simulink model "Scenario_13_CoDeSys"  (R2012b)
settings: Solver=ode3  StartTime=0.0  StopTime=inf  FixedStep=Sample_Time_Model  RelTol=1e-3
PreLoadFcn:
  | Variablen_Scenario13
InitFcn:
  | BT = randperm(9);
values from neighbouring files (symbols this model uses):
  Band_Geschwindigkeit = 1.47    [Variablen_Scenario13.m]
  Band_Sensor_Hell_2_Z = -6.5    [Variablen_Scenario13.m]
  Band_Sensor_Hell_3_Z = -10.36    [Variablen_Scenario13.m]
  Band_Sensor_Hell_4_Z = -14.64    [Variablen_Scenario13.m]
  Band_Sensor_Tolerance_Z = 0.2    [Variablen_Scenario13.m]
  Bauteil_Fallgeschwindigkeit = 0.4    [Variablen_Scenario13.m]
  Bauteil_Farbe_Metall = [0.8 0.8 0.8]    [Variablen_Scenario13.m]
  Bauteil_Farbe_Schwarz = [0.2 0.2 0.2]    [Variablen_Scenario13.m]
  Bauteil_Farbe_Weiss = [1 1 0.2]    [Variablen_Scenario13.m]
  Kran_Dauer_90_Grad = 5    [Variablen_Scenario13.m]
  Kran_Drehwinkel_90_Grad = 8050    [Variablen_Scenario13.m]
  Kran_Sensor_Position_Delta = 0.07    [Variablen_Scenario13.m]
  Sample_Time_Model = 0.05    [Variablen_Scenario13.m]
  Sample_Time_Simulation = 0.1    [Variablen_Scenario13.m]
  Sensor_Band_Metall_1 = -6.5    [Variablen_Scenario13.m]
  Sensor_Band_Metall_2 = -10.36    [Variablen_Scenario13.m]
libraries: simulink x557, vrlib x13, opclib x7, rtwinlib x1
(part 9 of 10)

== stateflow chart Scenario_13_CoDeSys/Signal Expander/Bauteil_3 ==
  state Stop1
  state Bauteil_3_Pos_2
  state Bauteil_2_Unten
  state Bauteil_3_Faellt_2
    during:
    BT_Y_Achse = Next_Pos_Minus_Min(BT_Y_Achse, Bauteil_Fallgeschwindigkeit, 0.7);
  state Drehen_Rechts_Runter [function]
    (default) -> (junction 322) : {BT_Y_Achse = Next_Pos_Minus_Min(BT_Y_Achse, Kran_Zyl_Schritt_Runter, 0.65);
        | x = x - Kran_Drehen_Schritt;
        | BT_Z_Achse = -3.5*sin(x);
        | BT_X_Achse = 3.5*cos(x);}
  state Drehen_Rechts_Hoch [function]
    (default) -> (junction 325) : {BT_Y_Achse = Next_Pos_Plus_Max(BT_Y_Achse, Kran_Zyl_Schritt_Hoch, 1.65);
        | x = x - Kran_Drehen_Schritt;
        | BT_Z_Achse = -3.5*sin(x);
        | BT_X_Achse = 3.5*cos(x);}
  state Bauteil_Lager_Vereinz_Ausfahren
    during:
    BT_X_Achse = BT_X_Achse - Lager_Vereinzler_Schritt_Aus;
  state Bauteil_Lager_Bereit
    entry: BT_Bereit = 1;
    BT_X_Achse = 3.5;
  state Drehen_Links_Runter [function]
    (default) -> (junction 319) : {BT_Y_Achse = Next_Pos_Minus_Min(BT_Y_Achse, Kran_Zyl_Schritt_Runter, 0.65);
        | x = x + Kran_Drehen_Schritt;
        | BT_Z_Achse = -3.5*sin(x);
        | BT_X_Achse = 3.5*cos(x);}
  state Drehen_Links_Hoch [function]
    (default) -> (junction 309) : {BT_Y_Achse = Next_Pos_Plus_Max(BT_Y_Achse, Kran_Zyl_Schritt_Hoch, 1.65);
        | x = x + Kran_Drehen_Schritt;
        | BT_Z_Achse = -3.5*sin(x);
        | BT_X_Achse = 3.5*cos(x);}
  state Ausgabe = Next_Pos_Plus_Max(Achse, Schrittgroesse, MaxWert) [function]
    (default) -> (junction 249) : {Naechste_Position = Achse + Schrittgroesse;}
    (junction 249) -> (junction 250) [order 1] : [Naechste_Position >= MaxWert]
    (junction 249) -> (junction 251) [order 2] : {Ausgabe = Naechste_Position;}
    (junction 250) -> (junction 252) : {Ausgabe = MaxWert;}
    (junction 252) -> (junction 251)
  state Bauteil_3_Pos_3
    entry:
    BT_X_Achse = 5.75;
    BT_Y_Achse = 2.72;
    x =0;
  state Bauteil_Kran_Hochheben_Bereit
    entry: BT_Bereit = 1;
    Kran_Sauger_BT = 1;
  state Bauteil_3_Faellt
    during:
    BT_Y_Achse = Next_Pos_Minus_Min(BT_Y_Achse, Bauteil_Fallgeschwindigkeit, 1.73);
  state Ausgabe = Next_Pos_Minus_Min(Achse, Schrittgroesse, MinWert) [function]
    (default) -> (junction 268) : {Naechste_Position = Achse - Schrittgroesse;}
    (junction 268) -> (junction 269) [order 1] : [Naechste_Position <= MinWert]
    (junction 268) -> (junction 270) [order 2] : {Ausgabe = Naechste_Position;}
    (junction 269) -> (junction 271) : {Ausgabe = MinWert;}
    (junction 271) -> (junction 270)
  state Ausgabe = Lager_Y_Achse(Lager_Status, Pos_1, Pos_2, Pos_3) [function]
    (default) -> (junction 374)
    (junction 374) -> (junction 373) [order 3] : [Lager_Status == 2]
    (junction 374) -> (junction 375) [order 1] : [Lager_Status == 0]
    (junction 373) -> (junction 376) : {Ausgabe = Pos_3;}
    (junction 374) -> (junction 377) [order 2] : [Lager_Status == 1]
        | {Ausgabe = Pos_2;}
    (junction 375) -> (junction 378) : {Ausgabe = Pos_1;}
    (junction 376) -> (junction 377)
    (junction 378) -> (junction 377)
  state Bauteil_Stempel_Halterung_Einfahren
    during:
    BT_X_Achse = Next_Pos_Minus_Min(BT_X_Achse, Stempel_Halterung_Schritt_Ein, -4.6);
  state Bauteil_Kran_Runterlassen
    during:
    BT_Y_Achse = Next_Pos_Minus_Min(BT_Y_Achse, Kran_Zyl_Schritt_Runter, 0.65);
  state Bauteil_Kran_Hochheben
    during:
    BT_Y_Achse = Next_Pos_Plus_Max(BT_Y_Achse, Kran_Zyl_Schritt_Hoch, 1.65);
  state Bauteil_Faellt_Auf_Festen_Untergrund
  state Bauteil_Lost
  state Bauteil_Lager_1_Ende
    entry: BT_Y_Achse = Lager_Y_Achse(Lager_1_Status, -0.158, 0.037, 0.232);
    BT_Lager = 1;
  state Bauteil_Abgesetzt_Stempel
    entry: Kran_Sauger_BT = 0;
  state Bauteil_Kran_Zyl_Stop
  state Bauteil_Stempel_Halterung_Stop
  state Drop_Down
    entry: Kran_Sauger_BT = 0;
    during:
    BT_Y_Achse = BT_Y_Achse - 0.4;
  state Bauteil_Lager_1_Beginnt
    entry: BT_Rotation_1 = 0;
    BT_Rotation_2 = 0;
    BT_Rotation_3 = 1;
    BT_Rotation_4 = 0.2;
    during:
    BT_X_Achse = Next_Pos_Minus_Min(BT_X_Achse, Band_Zyl_1_Schritt, -6.5 + Lager_1_Status);
    BT_Y_Achse = BT_Y_Achse - (0.2 * Band_Zyl_1_Schritt);
  state Bauteil_Stempel_Halterung_Ausfahren
    during:
    BT_X_Achse = Next_Pos_Plus_Max(BT_X_Achse, Stempel_Halterung_Schritt_Aus, -3.4);
  note: Bei -2,8 beginnt in etwa die Schraege !!
  state Drehen_Links
    during:
    x = x + Kran_Drehen_Schritt;
    BT_Z_Achse = -3.5*sin(x);
    BT_X_Achse = 3.5*cos(x);
  state Bauteil_Band_Vor
    during:
    BT_Z_Achse = BT_Z_Achse - Band_Geschwindigkeit;
  state Bauteil_Lager_1_Schieben
    during:
    BT_X_Achse = Next_Pos_Minus_Min(BT_X_Achse, Band_Zyl_1_Schritt, -2.7);
  state Bauteil_Lager_2_Ende
    entry: BT_Y_Achse = Lager_Y_Achse(Lager_2_Status, -0.158, 0.037, 0.232);
    BT_Lager = 2;
  state Bauteil_Kran_Rot_Stop
  state Bauteil_Band_Stop
    entry: Kran_Sauger_BT = 0;
  state Drehen_Rechts
    during:
    x = x - Kran_Drehen_Schritt;
    BT_Z_Achse = -3.5*sin(x);
    BT_X_Achse = 3.5*cos(x);
  state Bauteil_Lager_2_Beginnt
    entry: BT_Rotation_1 = 0;
    BT_Rotation_2 = 0;
    BT_Rotation_3 = 1;
    BT_Rotation_4 = 0.2;
    during:
    BT_X_Achse = Next_Pos_Minus_Min(BT_X_Achse, Band_Zyl_2_Schritt, -6.5 + Lager_2_Status);
    BT_Y_Achse = BT_Y_Achse - (0.2 * Band_Zyl_2_Schritt);
  state Bauteil_Band_Zurueck
    during:
    BT_Z_Achse = BT_Z_Achse + Band_Geschwindigkeit;
  state Bauteil_Lager_2_Schieben
    during:
    BT_X_Achse = Next_Pos_Minus_Min(BT_X_Achse, Band_Zyl_2_Schritt, -2.7);
  state Bauteil_Kran_Runterlassen_Und_Drehen_Rechts
    entry:
    x = x - Kran_Drehen_Schritt;
    BT_Z_Achse = -3.5*sin(x);
    BT_X_Achse = 3.5*cos(x);
    during: Drehen_Rechts_Runter();
  state Bauteil_Lager_3_Beginnt
    entry: BT_Rotation_1 = -1;
    BT_Rotation_2 = 0;
    BT_Rotation_3 = 0;
    BT_Rotation_4 = 0.2;
    during:
    BT_Z_Achse = Next_Pos_Minus_Min(BT_Z_Achse, 1.5 * Band_Geschwindigkeit, -19.05 + Lager_3_Status);
    BT_Y_Achse = BT_Y_Achse - (1.5 * 0.2*Band_Geschwindigkeit);
  state Bauteil_Kran_Hochheben_Und_Drehen_Links
    entry:
    x = x + Kran_Drehen_Schritt;
    BT_Z_Achse = -3.5*sin(x);
    BT_X_Achse = 3.5*cos(x);
    during: Drehen_Links_Hoch();
  state Bauteil_Lager_3_Ende
    entry: BT_Y_Achse = Lager_Y_Achse(Lager_3_Status, -0.158, 0.037, 0.232);
    BT_Lager = 3;
  state Bauteil_Kran_Hochheben_Und_Drehen_Rechts
    entry:
    x = x - Kran_Drehen_Schritt;
    BT_Z_Achse = -3.5*sin(x);
    BT_X_Achse = 3.5*cos(x);
    during:Drehen_Rechts_Hoch();
  state Bauteil_Kran_Runterlassen_Und_Drehen_Links
    entry:
    x = x + Kran_Drehen_Schritt;
    BT_Z_Achse = -3.5*sin(x);
    BT_X_Achse = 3.5*cos(x);
    during: Drehen_Links_Runter();
  Bauteil_Faellt_Auf_Festen_Untergrund -> Bauteil_Abgesetzt_Stempel [order 2] : [Kran_Stellung_Stempel]
  Stop1 -> Bauteil_Lager_Vereinz_Ausfahren : [BT_X_Achse + Lager_X_Achse >= 5.1]
  Bauteil_Lager_Vereinz_Ausfahren -> Stop1 [order 2] : [BT_X_Achse + Lager_X_Achse < 5.1]
  Bauteil_3_Pos_2 -> Bauteil_3_Faellt_2 : [BT_2_Bereit && Lager_Ver_Eingefahren]
  Bauteil_2_Unten -> Bauteil_Lager_Vereinz_Ausfahren : [Lager_Ver_Ausfahren && (BT_X_Achse + Lager_X_Achse >= 5.1)]
  Bauteil_3_Faellt -> Bauteil_3_Pos_2 : [BT_Y_Achse <= 1.73]
  Bauteil_3_Faellt_2 -> Bauteil_2_Unten : [BT_Y_Achse <= 0.7]
  Bauteil_Lager_Vereinz_Ausfahren -> Bauteil_Lager_Bereit [order 1] : [Lager_Ver_Ausgefahren]
  Bauteil_Faellt_Auf_Festen_Untergrund -> Bauteil_Lager_Bereit [order 1] : [Kran_Stellung_Lager]
  (default) -> Bauteil_3_Pos_3
  Bauteil_Lager_Bereit -> Bauteil_Kran_Hochheben_Bereit : [Kran_Stellung_Lager && Kran_Sauger && Kran_Zyl_Unten]
  Bauteil_Stempel_Halterung_Stop -> Bauteil_Kran_Hochheben_Bereit [order 3] : [Kran_Stellung_Stempel && Kran_Sauger && Kran_Zyl_Unten]
  (junction 127) -> Bauteil_Kran_Hochheben_Bereit [order 2] : [Kran_Stellung_Lager && Kran_Sauger && Kran_Zyl_Unten]
  Bauteil_Kran_Hochheben_Bereit -> Bauteil_Kran_Hochheben : [Kran_Hochheben]
      | {BT_Bereit = 0;}
  Bauteil_3_Pos_3 -> Bauteil_3_Faellt : [BT_1_Bereit && Lager_Ver_Eingefahren]
  Bauteil_Kran_Hochheben -> (junction 127) [order 3]
  Bauteil_Kran_Rot_Stop -> (junction 287) [order 4]
  (junction 287) -> Bauteil_Kran_Hochheben [order 2] : [Kran_Hochheben]
  (junction 287) -> Bauteil_Kran_Runterlassen [order 1] : [Kran_Runterlassen]
  Bauteil_Stempel_Halterung_Stop -> Bauteil_Stempel_Halterung_Einfahren [order 1] : [Stempel_Halterung_Einfahren]
  Bauteil_Stempel_Halterung_Einfahren -> Bauteil_Stempel_Halterung_Stop : [!Stempel_Halterung_Einfahren]
  Bauteil_Kran_Hochheben -> Bauteil_Kran_Runterlassen [order 1] : [Kran_Runterlassen]
  Bauteil_Kran_Runterlassen -> (junction 127) [order 2]
  Bauteil_Kran_Runterlassen -> (junction 162) [order 4]
  Bauteil_Kran_Zyl_Stop -> Bauteil_Kran_Runterlassen [order 3] : [Kran_Runterlassen]
  Bauteil_Kran_Runterlassen -> Bauteil_Kran_Zyl_Stop [order 3] : [Kran_Zyl_Unten]
  Bauteil_Kran_Runterlassen -> Bauteil_Kran_Hochheben [order 1] : [Kran_Hochheben]
  Drop_Down -> Bauteil_Faellt_Auf_Festen_Untergrund [order 2] : [(Kran_Stellung_Band || Kran_Stellung_Lager || Kran_Stellung_Stempel) && (BT_Y_Achse <= 0.65)]
  Drop_Down -> Bauteil_Lost [order 1] : [BT_Y_Achse <= -2]
  Bauteil_Kran_Hochheben -> (junction 162) [order 4]
  Bauteil_Kran_Hochheben -> Bauteil_Kran_Zyl_Stop [order 2] : [Kran_Zyl_Oben]
  Bauteil_Kran_Zyl_Stop -> Bauteil_Kran_Hochheben [order 2] : [Kran_Hochheben]
  Bauteil_Lager_1_Beginnt -> Bauteil_Lager_1_Ende : [BT_X_Achse <= (-6.5 + Lager_1_Status)]
  Bauteil_Abgesetzt_Stempel -> Bauteil_Stempel_Halterung_Stop
  Bauteil_Faellt_Auf_Festen_Untergrund -> Bauteil_Band_Stop [order 3] : [Kran_Stellung_Band]
  (junction 127) -> Drop_Down [order 1] : [!Kran_Sauger]
  Bauteil_Kran_Zyl_Stop -> (junction 127) [order 8]
  Bauteil_Kran_Zyl_Stop -> Bauteil_Abgesetzt_Stempel [order 6] : [Kran_Zyl_Unten && !Kran_Sauger && Kran_Stellung_Stempel]
  Drehen_Rechts -> Drop_Down [order 3] : [!Kran_Sauger]
  Bauteil_Stempel_Halterung_Ausfahren -> Bauteil_Stempel_Halterung_Stop : [!Stempel_Halterung_Ausfahren]
  Bauteil_Stempel_Halterung_Stop -> Bauteil_Stempel_Halterung_Ausfahren [order 2] : [Stempel_Halterung_Ausfahren]
  Bauteil_Kran_Rot_Stop -> Drop_Down [order 3] : [!Kran_Sauger]
  Drehen_Links -> Drop_Down [order 3] : [!Kran_Sauger]
  Bauteil_Kran_Zyl_Stop -> Drehen_Links [order 4] : [Kran_Drehen_Links]
  Bauteil_Kran_Zyl_Stop -> Drehen_Rechts [order 5] : [Kran_Drehen_Rechts]
  (junction 178) -> Bauteil_Kran_Zyl_Stop : [!Kran_Drehen_Rechts && !Kran_Drehen_Links]
  Bauteil_Kran_Zyl_Stop -> (junction 162) [order 1]
  Bauteil_Kran_Zyl_Stop -> Bauteil_Band_Stop [order 7] : [Kran_Zyl_Unten && !Kran_Sauger && Kran_Stellung_Band]
  Bauteil_Band_Stop -> Bauteil_Kran_Zyl_Stop [order 3] : [Kran_Zyl_Unten && Kran_Sauger && Kran_Stellung_Band && (-3.8 <= BT_Z_Achse) && (BT_Z_Achse <= -3.2) && (-0.5 <= BT_X_Achse) && (BT_X_Achse<= 0.5)]
  (junction 280) -> Drehen_Links [order 2] : [(Kran_Zyl_Unten || Kran_Zyl_Oben) && Kran_Drehen_Links]
      | {x = x + Kran_Drehen_Schritt;
      | BT_Z_Achse = -3.5*sin(x);
      | BT_X_Achse = 3.5*cos(x);}
  Drehen_Links -> Bauteil_Kran_Rot_Stop [order 2] : [!Kran_Drehen_Links]
  Bauteil_Lager_1_Schieben -> Bauteil_Lager_1_Beginnt : [BT_X_Achse <= -2.7]
  Bauteil_Kran_Rot_Stop -> Drehen_Links [order 1] : [Kran_Drehen_Links]
  Bauteil_Band_Vor -> (junction 135) [order 2]
  Drehen_Links -> (junction 162) [order 4]
  Drehen_Rechts -> Drehen_Links [order 1] : [Kran_Drehen_Links]
  Drehen_Links -> Drehen_Rechts [order 1] : [Kran_Drehen_Rechts]
  Bauteil_Band_Stop -> Bauteil_Band_Vor [order 1] : [Band_Vor]
  Bauteil_Band_Vor -> Bauteil_Band_Stop [order 1] : [!Band_Vor]
  (junction 135) -> Bauteil_Lager_1_Schieben [order 1] : [BT_Z_Achse <= -7.85 && BT_Z_Achse >= -8.65 && Band_Zyl_1_X_Achse >= -0.5]
  Bauteil_Lager_2_Beginnt -> Bauteil_Lager_2_Ende : [BT_X_Achse <= (-6.5 + Lager_2_Status)]
  (junction 280) -> Bauteil_Kran_Rot_Stop [order 3] : [Kran_Zyl_Unten || Kran_Zyl_Oben]
  Drehen_Rechts -> Bauteil_Kran_Rot_Stop [order 2] : [!Kran_Drehen_Rechts]
  Bauteil_Kran_Rot_Stop -> Drehen_Rechts [order 2] : [Kran_Drehen_Rechts]
  Bauteil_Band_Stop -> (junction 135) [order 4]
  (junction 135) -> Bauteil_Lager_2_Schieben [order 3] : [BT_Z_Achse <= -12.05 && BT_Z_Achse >= -12.85 && Band_Zyl_2_X_Achse >= -0.5]
  Bauteil_Band_Zurueck -> (junction 135) [order 2]
  (junction 135) -> Bauteil_Lager_3_Beginnt [order 2] : [BT_Z_Achse <= -14.6]
  Drehen_Rechts -> (junction 162) [order 4]
  Bauteil_Band_Zurueck -> Bauteil_Band_Stop [order 1] : [!Band_Zurueck]
  Bauteil_Band_Stop -> Bauteil_Band_Zurueck [order 2] : [Band_Zurueck]
  Bauteil_Kran_Runterlassen_Und_Drehen_Rechts -> (junction 178) [order 2]
  Bauteil_Kran_Hochheben_Und_Drehen_Links -> (junction 178) [order 2]
  Bauteil_Kran_Hochheben_Und_Drehen_Rechts -> (junction 178) [order 2]
  Bauteil_Kran_Runterlassen_Und_Drehen_Links -> (junction 178) [order 2]
  (junction 280) -> Drehen_Rechts [order 1] : [(Kran_Zyl_Unten || Kran_Zyl_Oben) && Kran_Drehen_Rechts]
      | {x = x - Kran_Drehen_Schritt;
      | BT_Z_Achse = -3.5*sin(x);
      | BT_X_Achse = 3.5*cos(x);}
  (junction 172) -> (junction 280)
  (junction 162) -> Bauteil_Kran_Runterlassen_Und_Drehen_Rechts [order 4] : [Kran_Drehen_Rechts && Kran_Runterlassen]
  (junction 162) -> Bauteil_Kran_Hochheben_Und_Drehen_Rechts [order 2] : [Kran_Drehen_Rechts && Kran_Hochheben]
  (junction 162) -> Bauteil_Kran_Hochheben_Und_Drehen_Links [order 1] : [Kran_Drehen_Links  && Kran_Hochheben]
  (junction 162) -> Bauteil_Kran_Runterlassen_Und_Drehen_Links [order 3] : [Kran_Drehen_Links  && Kran_Runterlassen]
  Bauteil_Lager_2_Schieben -> Bauteil_Lager_2_Beginnt : [BT_X_Achse <= -2.7]
  Bauteil_Kran_Runterlassen_Und_Drehen_Rechts -> (junction 172) [order 1]
  Bauteil_Lager_3_Beginnt -> Bauteil_Lager_3_Ende : [BT_Z_Achse <= (-19.05 + Lager_3_Status)]
  Bauteil_Kran_Hochheben_Und_Drehen_Rechts -> Bauteil_Kran_Runterlassen_Und_Drehen_Rechts [order 3] : [Kran_Drehen_Rechts  && Kran_Runterlassen]
  Bauteil_Kran_Runterlassen_Und_Drehen_Rechts -> Bauteil_Kran_Hochheben_Und_Drehen_Rechts [order 3] : [Kran_Drehen_Rechts  && Kran_Hochheben]
  Bauteil_Kran_Hochheben_Und_Drehen_Rechts -> (junction 172) [order 1]
  Bauteil_Kran_Hochheben_Und_Drehen_Links -> (junction 172) [order 1]
  Bauteil_Kran_Hochheben_Und_Drehen_Links -> Bauteil_Kran_Runterlassen_Und_Drehen_Links [order 3] : [Kran_Drehen_Links  && Kran_Runterlassen]
  Bauteil_Kran_Runterlassen_Und_Drehen_Links -> Bauteil_Kran_Hochheben_Und_Drehen_Links [order 3] : [Kran_Drehen_Links  && Kran_Hochheben]
  Bauteil_Kran_Runterlassen_Und_Drehen_Links -> (junction 172) [order 1]
  data: Achse function_input double; Schrittgroesse function_input double; MaxWert function_input double; Ausgabe function_output double; Achse function_input double; Schrittgroesse function_input double; MinWert function_input double; Ausgabe function_output double; Lager_Status function_input double; Pos_1 function_input double; Pos_2 function_input double; Ausgabe function_output double; Pos_3 function_input double; BT_Y_Achse output double; BT_Lager output double; Kran_Sauger_BT output double; BT_Bereit output double; BT_X_Achse output double; BT_Z_Achse output double; x local double; Lager_X_Achse input; Lager_Ver_Eingefahren input; Lager_Ver_Ausgefahren input; Kran_Stellung_Lager input; Kran_Stellung_Band input; Kran_Stellung_Stempel input; Kran_Zyl_Oben input; Kran_Zyl_Unten input; Kran_Sauger input; Kran_Hochheben input; Kran_Runterlassen input; Kran_Drehen_Links input; Kran_Drehen_Rechts input; Stempel_Halterung_Ausfahren input; Stempel_Halterung_Einfahren input; Band_Vor input; Band_Zurueck input; Band_Zyl_1_X_Achse input; Band_Zyl_2_X_Achse input; BT_Rotation_1 output double; BT_Rotation_2 output double; BT_Rotation_3 output double; BT_Rotation_4 output double; Lager_Ver_Ausfahren input; Lager_Vereinzler_Schritt_Aus input; Kran_Zyl_Schritt_Hoch input; Kran_Zyl_Schritt_Runter input; Kran_Drehen_Schritt input; Stempel_Halterung_Schritt_Aus input; Stempel_Halterung_Schritt_Ein input; Band_Zyl_1_Schritt input; Band_Zyl_2_Schritt input double; Band_Geschwindigkeit input; Bauteil_Fallgeschwindigkeit input double; Lager_1_Status input; Lager_2_Status input; Lager_3_Status input; Naechste_Position local double; BT_1_Bereit input; BT_2_Bereit input

== system Scenario_13_CoDeSys/Signal Expander/Subsystem1 ==
  Notaus_Knopf : Inport
  BT_Y_In : Inport  Port=2
  BT_Lager_In : Inport  Port=3
  BT_angesaugt_in : Inport  Port=4
  BT_Bereit : Inport  Port=5
  Add : Sum  Inputs=-+
  Compare To Constant : simulink/Logic and Bit Operations/Compare To Constant  relop===  const=0  OutDataTypeStr=boolean
  Constant : Constant  Value=5000
  Constant1 : Constant  Value=0
  Constant2 : Constant  Value=0
  Constant3 : Constant  Value=0
  Detect Decrease : simulink/Logic and Bit Operations/Detect Decrease  vinit=0.0  InputProcessing=Inherited  OutDataTypeStr=boolean
  Logical Operator : Logic  Operator=OR  AllPortsSameDT=off  OutDataTypeStr=boolean
  Logical Operator1 : Logic  Inputs=3  AllPortsSameDT=off  OutDataTypeStr=boolean
  Logical Operator2 : Logic  Operator=OR  AllPortsSameDT=off  OutDataTypeStr=boolean
  Memory : Memory
  Memory1 : Memory
  Switch{,1..3} (4 alike) : Switch  Threshold=1
  BT_Y_Out : Outport
  BT_Angesaugt_Out : Outport  Port=2
  BT_Lager_Out : Outport  Port=3
  BT_Bereit_Out : Outport  Port=4
  wires:
  BT_Bereit/1 -> Switch3/3, Logical Operator/1
  Memory/1 -> Logical Operator/2
  BT_Y_In/1 -> Switch/3, Add/2
  Compare To Constant/1 -> Logical Operator1/1
  Logical Operator/1 -> Memory/1, Logical Operator1/2
  Constant/1 -> Add/1
  Add/1 -> Switch/1
  Switch/1 -> BT_Y_Out/1
  Notaus_Knopf/1 -> Detect Decrease/1
  Detect Decrease/1 -> Logical Operator1/3
  Logical Operator1/1 -> Logical Operator2/1
  Memory1/1 -> Logical Operator2/2
  Logical Operator2/1 -> Switch1/2, Switch3/2, Switch2/2, Switch/2, Memory1/1
  BT_angesaugt_in/1 -> Switch1/3
  Constant1/1 -> Switch1/1
  Switch1/1 -> BT_Angesaugt_Out/1
  BT_Lager_In/1 -> Switch2/3, Compare To Constant/1
  Constant2/1 -> Switch2/1
  Switch2/1 -> BT_Lager_Out/1
  Constant3/1 -> Switch3/1
  Switch3/1 -> BT_Bereit_Out/1

== system Scenario_13_CoDeSys/Signal Expander/Subsystem2 ==
  Notaus_Knopf : Inport
  BT_Y_In : Inport  Port=2
  BT_Lager_In : Inport  Port=3
  BT_angesaugt_in : Inport  Port=4
  BT_Bereit : Inport  Port=5
  Add : Sum  Inputs=-+
  Compare To Constant : simulink/Logic and Bit Operations/Compare To Constant  relop===  const=0  OutDataTypeStr=boolean
  Constant : Constant  Value=5000
  Constant1 : Constant  Value=0
  Constant2 : Constant  Value=0
  Constant3 : Constant  Value=0
  Detect Decrease : simulink/Logic and Bit Operations/Detect Decrease  vinit=0.0  InputProcessing=Inherited  OutDataTypeStr=boolean
  Logical Operator : Logic  Operator=OR  AllPortsSameDT=off  OutDataTypeStr=boolean
  Logical Operator1 : Logic  Inputs=3  AllPortsSameDT=off  OutDataTypeStr=boolean
  Logical Operator2 : Logic  Operator=OR  AllPortsSameDT=off  OutDataTypeStr=boolean
  Memory : Memory
  Memory1 : Memory
  Switch{,1..3} (4 alike) : Switch  Threshold=1
  BT_Y_Out : Outport
  BT_Angesaugt_Out : Outport  Port=2
  BT_Lager_Out : Outport  Port=3
  BT_Bereit_Out : Outport  Port=4
  wires:
  BT_Bereit/1 -> Switch3/3, Logical Operator/1
  Memory/1 -> Logical Operator/2
  BT_Y_In/1 -> Switch/3, Add/2
  Compare To Constant/1 -> Logical Operator1/1
  Logical Operator/1 -> Memory/1, Logical Operator1/2
  Constant/1 -> Add/1
  Add/1 -> Switch/1
  Switch/1 -> BT_Y_Out/1
  Notaus_Knopf/1 -> Detect Decrease/1
  Detect Decrease/1 -> Logical Operator1/3
  Logical Operator1/1 -> Logical Operator2/1
  Memory1/1 -> Logical Operator2/2
  Logical Operator2/1 -> Switch1/2, Switch3/2, Switch2/2, Switch/2, Memory1/1
  BT_angesaugt_in/1 -> Switch1/3
  Constant1/1 -> Switch1/1
  Switch1/1 -> BT_Angesaugt_Out/1
  BT_Lager_In/1 -> Switch2/3, Compare To Constant/1
  Constant2/1 -> Switch2/1
  Switch2/1 -> BT_Lager_Out/1
  Constant3/1 -> Switch3/1
  Switch3/1 -> BT_Bereit_Out/1

== system Scenario_13_CoDeSys/Signal Expander/Subsystem3 ==
  Notaus_Knopf : Inport
  BT_Y_In : Inport  Port=2
  BT_Lager_In : Inport  Port=3
  BT_angesaugt_in : Inport  Port=4
  BT_Bereit : Inport  Port=5
  Add : Sum  Inputs=-+
  Compare To Constant : simulink/Logic and Bit Operations/Compare To Constant  relop===  const=0  OutDataTypeStr=boolean
  Constant : Constant  Value=5000
  Constant1 : Constant  Value=0
  Constant2 : Constant  Value=0
  Constant3 : Constant  Value=0
  Detect Decrease : simulink/Logic and Bit Operations/Detect Decrease  vinit=0.0  InputProcessing=Inherited  OutDataTypeStr=boolean
  Logical Operator : Logic  Operator=OR  AllPortsSameDT=off  OutDataTypeStr=boolean
  Logical Operator1 : Logic  Inputs=3  AllPortsSameDT=off  OutDataTypeStr=boolean
  Logical Operator2 : Logic  Operator=OR  AllPortsSameDT=off  OutDataTypeStr=boolean
  Memory : Memory
  Memory1 : Memory
  Switch{,1..3} (4 alike) : Switch  Threshold=1
  BT_Y_Out : Outport
  BT_Angesaugt_Out : Outport  Port=2
  BT_Lager_Out : Outport  Port=3
  BT_Bereit_Out : Outport  Port=4
  wires:
  BT_Bereit/1 -> Switch3/3, Logical Operator/1
  Memory/1 -> Logical Operator/2
  BT_Y_In/1 -> Switch/3, Add/2
  Compare To Constant/1 -> Logical Operator1/1
  Logical Operator/1 -> Memory/1, Logical Operator1/2
  Constant/1 -> Add/1
  Add/1 -> Switch/1
  Switch/1 -> BT_Y_Out/1
  Notaus_Knopf/1 -> Detect Decrease/1
  Detect Decrease/1 -> Logical Operator1/3
  Logical Operator1/1 -> Logical Operator2/1
  Memory1/1 -> Logical Operator2/2
  Logical Operator2/1 -> Switch1/2, Switch3/2, Switch2/2, Switch/2, Memory1/1
  BT_angesaugt_in/1 -> Switch1/3
  Constant1/1 -> Switch1/1
  Switch1/1 -> BT_Angesaugt_Out/1
  BT_Lager_In/1 -> Switch2/3, Compare To Constant/1
  Constant2/1 -> Switch2/1
  Switch2/1 -> BT_Lager_Out/1
  Constant3/1 -> Switch3/1
  Switch3/1 -> BT_Bereit_Out/1

== system Scenario_13_CoDeSys/Signal Expander/Subsystem4 ==
  Notaus_Knopf : Inport
  BT_Y_In : Inport  Port=2
  BT_Lager_In : Inport  Port=3
  BT_angesaugt_in : Inport  Port=4
  BT_Bereit : Inport  Port=5
  Add : Sum  Inputs=-+
  Compare To Constant : simulink/Logic and Bit Operations/Compare To Constant  relop===  const=0  OutDataTypeStr=boolean
  Constant : Constant  Value=5000
  Constant1 : Constant  Value=0
  Constant2 : Constant  Value=0
  Constant3 : Constant  Value=0
  Detect Decrease : simulink/Logic and Bit Operations/Detect Decrease  vinit=0.0  InputProcessing=Inherited  OutDataTypeStr=boolean
  Logical Operator : Logic  Operator=OR  AllPortsSameDT=off  OutDataTypeStr=boolean
  Logical Operator1 : Logic  Inputs=3  AllPortsSameDT=off  OutDataTypeStr=boolean
  Logical Operator2 : Logic  Operator=OR  AllPortsSameDT=off  OutDataTypeStr=boolean
  Memory : Memory
  Memory1 : Memory
  Switch{,1..3} (4 alike) : Switch  Threshold=1
  BT_Y_Out : Outport
  BT_Angesaugt_Out : Outport  Port=2
  BT_Lager_Out : Outport  Port=3
  BT_Bereit_Out : Outport  Port=4
  wires:
  BT_Bereit/1 -> Switch3/3, Logical Operator/1
  Memory/1 -> Logical Operator/2
  BT_Y_In/1 -> Switch/3, Add/2
  Compare To Constant/1 -> Logical Operator1/1
  Logical Operator/1 -> Memory/1, Logical Operator1/2
  Constant/1 -> Add/1
  Add/1 -> Switch/1
  Switch/1 -> BT_Y_Out/1
  Notaus_Knopf/1 -> Detect Decrease/1
  Detect Decrease/1 -> Logical Operator1/3
  Logical Operator1/1 -> Logical Operator2/1
  Memory1/1 -> Logical Operator2/2
  Logical Operator2/1 -> Switch1/2, Switch3/2, Switch2/2, Switch/2, Memory1/1
  BT_angesaugt_in/1 -> Switch1/3
  Constant1/1 -> Switch1/1
  Switch1/1 -> BT_Angesaugt_Out/1
  BT_Lager_In/1 -> Switch2/3, Compare To Constant/1
  Constant2/1 -> Switch2/1
  Switch2/1 -> BT_Lager_Out/1
  Constant3/1 -> Switch3/1
  Switch3/1 -> BT_Bereit_Out/1

== system Scenario_13_CoDeSys/Signal Expander/Subsystem5 ==
  Notaus_Knopf : Inport
  BT_Y_In : Inport  Port=2
  BT_Lager_In : Inport  Port=3
  BT_angesaugt_in : Inport  Port=4
  BT_Bereit : Inport  Port=5
  Add : Sum  Inputs=-+
  Compare To Constant : simulink/Logic and Bit Operations/Compare To Constant  relop===  const=0  OutDataTypeStr=boolean
  Constant : Constant  Value=5000
  Constant1 : Constant  Value=0
  Constant2 : Constant  Value=0
  Constant3 : Constant  Value=0
  Detect Decrease : simulink/Logic and Bit Operations/Detect Decrease  vinit=0.0  InputProcessing=Inherited  OutDataTypeStr=boolean
  Logical Operator : Logic  Operator=OR  AllPortsSameDT=off  OutDataTypeStr=boolean
  Logical Operator1 : Logic  Inputs=3  AllPortsSameDT=off  OutDataTypeStr=boolean
  Logical Operator2 : Logic  Operator=OR  AllPortsSameDT=off  OutDataTypeStr=boolean
  Memory : Memory
  Memory1 : Memory
  Switch{,1..3} (4 alike) : Switch  Threshold=1
  BT_Y_Out : Outport
  BT_Angesaugt_Out : Outport  Port=2
  BT_Lager_Out : Outport  Port=3
  BT_Bereit_Out : Outport  Port=4
  wires:
  BT_Bereit/1 -> Switch3/3, Logical Operator/1
  Memory/1 -> Logical Operator/2
  BT_Y_In/1 -> Switch/3, Add/2
  Compare To Constant/1 -> Logical Operator1/1
  Logical Operator/1 -> Memory/1, Logical Operator1/2
  Constant/1 -> Add/1
  Add/1 -> Switch/1
  Switch/1 -> BT_Y_Out/1
  Notaus_Knopf/1 -> Detect Decrease/1
  Detect Decrease/1 -> Logical Operator1/3
  Logical Operator1/1 -> Logical Operator2/1
  Memory1/1 -> Logical Operator2/2
  Logical Operator2/1 -> Switch1/2, Switch3/2, Switch2/2, Switch/2, Memory1/1
  BT_angesaugt_in/1 -> Switch1/3
  Constant1/1 -> Switch1/1
  Switch1/1 -> BT_Angesaugt_Out/1
  BT_Lager_In/1 -> Switch2/3, Compare To Constant/1
  Constant2/1 -> Switch2/1
  Switch2/1 -> BT_Lager_Out/1
  Constant3/1 -> Switch3/1
  Switch3/1 -> BT_Bereit_Out/1

== system Scenario_13_CoDeSys/Signal Expander/Subsystem6 ==
  Notaus_Knopf : Inport
  BT_Y_In : Inport  Port=2
  BT_Lager_In : Inport  Port=3
  BT_angesaugt_in : Inport  Port=4
  BT_Bereit : Inport  Port=5
  Add : Sum  Inputs=-+
  Compare To Constant : simulink/Logic and Bit Operations/Compare To Constant  relop===  const=0  OutDataTypeStr=boolean
  Constant : Constant  Value=5000
  Constant1 : Constant  Value=0
  Constant2 : Constant  Value=0
  Constant3 : Constant  Value=0
  Detect Decrease : simulink/Logic and Bit Operations/Detect Decrease  vinit=0.0  InputProcessing=Inherited  OutDataTypeStr=boolean
  Logical Operator : Logic  Operator=OR  AllPortsSameDT=off  OutDataTypeStr=boolean
  Logical Operator1 : Logic  Inputs=3  AllPortsSameDT=off  OutDataTypeStr=boolean
  Logical Operator2 : Logic  Operator=OR  AllPortsSameDT=off  OutDataTypeStr=boolean
  Memory : Memory
  Memory1 : Memory
  Switch{,1..3} (4 alike) : Switch  Threshold=1
  BT_Y_Out : Outport
  BT_Angesaugt_Out : Outport  Port=2
  BT_Lager_Out : Outport  Port=3
  BT_Bereit_Out : Outport  Port=4
  wires:
  BT_Bereit/1 -> Switch3/3, Logical Operator/1
  Memory/1 -> Logical Operator/2
  BT_Y_In/1 -> Switch/3, Add/2
  Compare To Constant/1 -> Logical Operator1/1
  Logical Operator/1 -> Memory/1, Logical Operator1/2
  Constant/1 -> Add/1
  Add/1 -> Switch/1
  Switch/1 -> BT_Y_Out/1
  Notaus_Knopf/1 -> Detect Decrease/1
  Detect Decrease/1 -> Logical Operator1/3
  Logical Operator1/1 -> Logical Operator2/1
  Memory1/1 -> Logical Operator2/2
  Logical Operator2/1 -> Switch1/2, Switch3/2, Switch2/2, Switch/2, Memory1/1
  BT_angesaugt_in/1 -> Switch1/3
  Constant1/1 -> Switch1/1
  Switch1/1 -> BT_Angesaugt_Out/1
  BT_Lager_In/1 -> Switch2/3, Compare To Constant/1
  Constant2/1 -> Switch2/1
  Switch2/1 -> BT_Lager_Out/1
  Constant3/1 -> Switch3/1
  Switch3/1 -> BT_Bereit_Out/1

== system Scenario_13_CoDeSys/Signal Expander/Subsystem7 ==
  Notaus_Knopf : Inport
  BT_Y_In : Inport  Port=2
  BT_Lager_In : Inport  Port=3
  BT_angesaugt_in : Inport  Port=4
  BT_Bereit : Inport  Port=5
  Add : Sum  Inputs=-+
  Compare To Constant : simulink/Logic and Bit Operations/Compare To Constant  relop===  const=0  OutDataTypeStr=boolean
  Constant : Constant  Value=5000
  Constant1 : Constant  Value=0
  Constant2 : Constant  Value=0
  Constant3 : Constant  Value=0
  Detect Decrease : simulink/Logic and Bit Operations/Detect Decrease  vinit=0.0  InputProcessing=Inherited  OutDataTypeStr=boolean
  Logical Operator : Logic  Operator=OR  AllPortsSameDT=off  OutDataTypeStr=boolean
  Logical Operator1 : Logic  Inputs=3  AllPortsSameDT=off  OutDataTypeStr=boolean
  Logical Operator2 : Logic  Operator=OR  AllPortsSameDT=off  OutDataTypeStr=boolean
  Memory : Memory
  Memory1 : Memory
  Switch{,1..3} (4 alike) : Switch  Threshold=1
  BT_Y_Out : Outport
  BT_Angesaugt_Out : Outport  Port=2
  BT_Lager_Out : Outport  Port=3
  BT_Bereit_Out : Outport  Port=4
  wires:
  BT_Bereit/1 -> Switch3/3, Logical Operator/1
  Memory/1 -> Logical Operator/2
  BT_Y_In/1 -> Switch/3, Add/2
  Compare To Constant/1 -> Logical Operator1/1
  Logical Operator/1 -> Memory/1, Logical Operator1/2
  Constant/1 -> Add/1
  Add/1 -> Switch/1
  Switch/1 -> BT_Y_Out/1
  Notaus_Knopf/1 -> Detect Decrease/1
  Detect Decrease/1 -> Logical Operator1/3
  Logical Operator1/1 -> Logical Operator2/1
  Memory1/1 -> Logical Operator2/2
  Logical Operator2/1 -> Switch1/2, Switch3/2, Switch2/2, Switch/2, Memory1/1
  BT_angesaugt_in/1 -> Switch1/3
  Constant1/1 -> Switch1/1
  Switch1/1 -> BT_Angesaugt_Out/1
  BT_Lager_In/1 -> Switch2/3, Compare To Constant/1
  Constant2/1 -> Switch2/1
  Switch2/1 -> BT_Lager_Out/1
  Constant3/1 -> Switch3/1
  Switch3/1 -> BT_Bereit_Out/1

== system Scenario_13_CoDeSys/Signal Expander/Subsystem8 ==
  Notaus_Knopf : Inport
  BT_Y_In : Inport  Port=2
  BT_Lager_In : Inport  Port=3
  BT_angesaugt_in : Inport  Port=4
  BT_Bereit : Inport  Port=5
  Add : Sum  Inputs=-+
  Compare To Constant : simulink/Logic and Bit Operations/Compare To Constant  relop===  const=0  OutDataTypeStr=boolean
  Constant : Constant  Value=5000
  Constant1 : Constant  Value=0
  Constant2 : Constant  Value=0
  Constant3 : Constant  Value=0
  Detect Decrease : simulink/Logic and Bit Operations/Detect Decrease  vinit=0.0  InputProcessing=Inherited  OutDataTypeStr=boolean
  Logical Operator : Logic  Operator=OR  AllPortsSameDT=off  OutDataTypeStr=boolean
  Logical Operator1 : Logic  Inputs=3  AllPortsSameDT=off  OutDataTypeStr=boolean
  Logical Operator2 : Logic  Operator=OR  AllPortsSameDT=off  OutDataTypeStr=boolean
  Memory : Memory
  Memory1 : Memory
  Switch{,1..3} (4 alike) : Switch  Threshold=1
  BT_Y_Out : Outport
  BT_Angesaugt_Out : Outport  Port=2
  BT_Lager_Out : Outport  Port=3
  BT_Bereit_Out : Outport  Port=4
  wires:
  BT_Bereit/1 -> Switch3/3, Logical Operator/1
  Memory/1 -> Logical Operator/2
  BT_Y_In/1 -> Switch/3, Add/2
  Compare To Constant/1 -> Logical Operator1/1
  Logical Operator/1 -> Memory/1, Logical Operator1/2
  Constant/1 -> Add/1
  Add/1 -> Switch/1
  Switch/1 -> BT_Y_Out/1
  Notaus_Knopf/1 -> Detect Decrease/1
  Detect Decrease/1 -> Logical Operator1/3
  Logical Operator1/1 -> Logical Operator2/1
  Memory1/1 -> Logical Operator2/2
  Logical Operator2/1 -> Switch1/2, Switch3/2, Switch2/2, Switch/2, Memory1/1
  BT_angesaugt_in/1 -> Switch1/3
  Constant1/1 -> Switch1/1
  Switch1/1 -> BT_Angesaugt_Out/1
  BT_Lager_In/1 -> Switch2/3, Compare To Constant/1
  Constant2/1 -> Switch2/1
  Switch2/1 -> BT_Lager_Out/1
  Constant3/1 -> Switch3/1
  Switch3/1 -> BT_Bereit_Out/1

== system Scenario_13_CoDeSys/Stempelanlage/BT_2_Farbe ==
  In : Inport
  Compare To Constant : simulink/Logic and Bit Operations/Compare To Constant  relop===  const=0  OutDataTypeStr=boolean
  Compare To Constant1 : simulink/Logic and Bit Operations/Compare To Constant  relop===  const=1  OutDataTypeStr=boolean
  Compare To Constant2 : simulink/Logic and Bit Operations/Compare To Constant  relop===  const=2  OutDataTypeStr=boolean
  Constant : Constant  Value=[0 0 0]
  Constant1 : Constant  Value=[0 0 0]
  Constant2 : Constant  Value=[0 0 0]
  Metall : Constant  Value=Bauteil_Farbe_Metall
  MinMax : MinMax  Function=max  Inputs=3
  Schwarz : Constant  Value=Bauteil_Farbe_Schwarz
  Switch : Switch  Threshold=1
  Switch1 : Switch  Threshold=1
  Switch2 : Switch  Threshold=1
  Weiss(Gelb) : Constant  Value=Bauteil_Farbe_Weiss
  Out : Outport
  wires:
  In/1 -> Compare To Constant1/1, Compare To Constant2/1, Compare To Constant/1
  Compare To Constant1/1 -> Switch/2
  Compare To Constant/1 -> Switch2/2
  Compare To Constant2/1 -> Switch1/2
  Metall/1 -> Switch1/1
  Schwarz/1 -> Switch/1
  Weiss(Gelb)/1 -> Switch2/1
  Constant/1 -> Switch2/3
  Constant2/1 -> Switch/3
  Constant1/1 -> Switch1/3
  Switch/1 -> MinMax/2
  Switch2/1 -> MinMax/1
  Switch1/1 -> MinMax/3
  MinMax/1 -> Out/1

== system Scenario_13_CoDeSys/Stempelanlage/BT_2_Farbe1 ==
  In : Inport
  Compare To Constant : simulink/Logic and Bit Operations/Compare To Constant  relop===  const=0  OutDataTypeStr=boolean
  Compare To Constant1 : simulink/Logic and Bit Operations/Compare To Constant  relop===  const=1  OutDataTypeStr=boolean
  Compare To Constant2 : simulink/Logic and Bit Operations/Compare To Constant  relop===  const=2  OutDataTypeStr=boolean
  Constant : Constant  Value=[0 0 0]
  Constant1 : Constant  Value=[0 0 0]
  Constant2 : Constant  Value=[0 0 0]
  Metall : Constant  Value=Bauteil_Farbe_Metall
  MinMax : MinMax  Function=max  Inputs=3
  Schwarz : Constant  Value=Bauteil_Farbe_Schwarz
  Switch : Switch  Threshold=1
  Switch1 : Switch  Threshold=1
  Switch2 : Switch  Threshold=1
  Weiss(Gelb) : Constant  Value=Bauteil_Farbe_Weiss
  Out : Outport
  wires:
  In/1 -> Compare To Constant1/1, Compare To Constant2/1, Compare To Constant/1
  Compare To Constant1/1 -> Switch/2
  Compare To Constant/1 -> Switch2/2
  Compare To Constant2/1 -> Switch1/2
  Metall/1 -> Switch1/1
  Schwarz/1 -> Switch/1
  Weiss(Gelb)/1 -> Switch2/1
  Constant/1 -> Switch2/3
  Constant2/1 -> Switch/3
  Constant1/1 -> Switch1/3
  Switch/1 -> MinMax/2
  Switch2/1 -> MinMax/1
  Switch1/1 -> MinMax/3
  MinMax/1 -> Out/1

== system Scenario_13_CoDeSys/Stempelanlage/BT_3_Farbe ==
  In : Inport
  Compare To Constant : simulink/Logic and Bit Operations/Compare To Constant  relop===  const=0  OutDataTypeStr=boolean
  Compare To Constant1 : simulink/Logic and Bit Operations/Compare To Constant  relop===  const=1  OutDataTypeStr=boolean
  Compare To Constant2 : simulink/Logic and Bit Operations/Compare To Constant  relop===  const=2  OutDataTypeStr=boolean
  Constant : Constant  Value=[0 0 0]
  Constant1 : Constant  Value=[0 0 0]
  Constant2 : Constant  Value=[0 0 0]
  Metall : Constant  Value=Bauteil_Farbe_Metall
  MinMax : MinMax  Function=max  Inputs=3
  Schwarz : Constant  Value=Bauteil_Farbe_Schwarz
  Switch : Switch  Threshold=1
  Switch1 : Switch  Threshold=1
  Switch2 : Switch  Threshold=1
  Weiss(Gelb) : Constant  Value=Bauteil_Farbe_Weiss
  Out : Outport
  wires:
  In/1 -> Compare To Constant1/1, Compare To Constant2/1, Compare To Constant/1
  Compare To Constant1/1 -> Switch/2
  Compare To Constant/1 -> Switch2/2
  Compare To Constant2/1 -> Switch1/2
  Metall/1 -> Switch1/1
  Schwarz/1 -> Switch/1
  Weiss(Gelb)/1 -> Switch2/1
  Constant/1 -> Switch2/3
  Constant2/1 -> Switch/3
  Constant1/1 -> Switch1/3
  Switch/1 -> MinMax/2
  Switch2/1 -> MinMax/1
  Switch1/1 -> MinMax/3
  MinMax/1 -> Out/1

== system Scenario_13_CoDeSys/Stempelanlage/BT_4_Farbe ==
  In : Inport
  Compare To Constant : simulink/Logic and Bit Operations/Compare To Constant  relop===  const=0  OutDataTypeStr=boolean
  Compare To Constant1 : simulink/Logic and Bit Operations/Compare To Constant  relop===  const=1  OutDataTypeStr=boolean
  Compare To Constant2 : simulink/Logic and Bit Operations/Compare To Constant  relop===  const=2  OutDataTypeStr=boolean
  Constant : Constant  Value=[0 0 0]
  Constant1 : Constant  Value=[0 0 0]
  Constant2 : Constant  Value=[0 0 0]
  Metall : Constant  Value=Bauteil_Farbe_Metall
  MinMax : MinMax  Function=max  Inputs=3
  Schwarz : Constant  Value=Bauteil_Farbe_Schwarz
  Switch : Switch  Threshold=1
  Switch1 : Switch  Threshold=1
  Switch2 : Switch  Threshold=1
  Weiss(Gelb) : Constant  Value=Bauteil_Farbe_Weiss
  Out : Outport
  wires:
  In/1 -> Compare To Constant1/1, Compare To Constant2/1, Compare To Constant/1
  Compare To Constant1/1 -> Switch/2
  Compare To Constant/1 -> Switch2/2
  Compare To Constant2/1 -> Switch1/2
  Metall/1 -> Switch1/1
  Schwarz/1 -> Switch/1
  Weiss(Gelb)/1 -> Switch2/1
  Constant/1 -> Switch2/3
  Constant2/1 -> Switch/3
  Constant1/1 -> Switch1/3
  Switch/1 -> MinMax/2
  Switch2/1 -> MinMax/1
  Switch1/1 -> MinMax/3
  MinMax/1 -> Out/1

== system Scenario_13_CoDeSys/Stempelanlage/BT_5_Farbe ==
  In : Inport
  Compare To Constant : simulink/Logic and Bit Operations/Compare To Constant  relop===  const=0  OutDataTypeStr=boolean
  Compare To Constant1 : simulink/Logic and Bit Operations/Compare To Constant  relop===  const=1  OutDataTypeStr=boolean
  Compare To Constant2 : simulink/Logic and Bit Operations/Compare To Constant  relop===  const=2  OutDataTypeStr=boolean
  Constant : Constant  Value=[0 0 0]
  Constant1 : Constant  Value=[0 0 0]
  Constant2 : Constant  Value=[0 0 0]
  Metall : Constant  Value=Bauteil_Farbe_Metall
  MinMax : MinMax  Function=max  Inputs=3
  Schwarz : Constant  Value=Bauteil_Farbe_Schwarz
  Switch : Switch  Threshold=1
  Switch1 : Switch  Threshold=1
  Switch2 : Switch  Threshold=1
  Weiss(Gelb) : Constant  Value=Bauteil_Farbe_Weiss
  Out : Outport
  wires:
  In/1 -> Compare To Constant1/1, Compare To Constant2/1, Compare To Constant/1
  Compare To Constant1/1 -> Switch/2
  Compare To Constant/1 -> Switch2/2
  Compare To Constant2/1 -> Switch1/2
  Metall/1 -> Switch1/1
  Schwarz/1 -> Switch/1
  Weiss(Gelb)/1 -> Switch2/1
  Constant/1 -> Switch2/3
  Constant2/1 -> Switch/3
  Constant1/1 -> Switch1/3
  Switch/1 -> MinMax/2
  Switch2/1 -> MinMax/1
  Switch1/1 -> MinMax/3
  MinMax/1 -> Out/1

== system Scenario_13_CoDeSys/Stempelanlage/BT_6_Farbe ==
  In : Inport
  Compare To Constant : simulink/Logic and Bit Operations/Compare To Constant  relop===  const=0  OutDataTypeStr=boolean
  Compare To Constant1 : simulink/Logic and Bit Operations/Compare To Constant  relop===  const=1  OutDataTypeStr=boolean
  Compare To Constant2 : simulink/Logic and Bit Operations/Compare To Constant  relop===  const=2  OutDataTypeStr=boolean
  Constant : Constant  Value=[0 0 0]
  Constant1 : Constant  Value=[0 0 0]
  Constant2 : Constant  Value=[0 0 0]
  Metall : Constant  Value=Bauteil_Farbe_Metall
  MinMax : MinMax  Function=max  Inputs=3
  Schwarz : Constant  Value=Bauteil_Farbe_Schwarz
  Switch : Switch  Threshold=1
  Switch1 : Switch  Threshold=1
  Switch2 : Switch  Threshold=1
  Weiss(Gelb) : Constant  Value=Bauteil_Farbe_Weiss
  Out : Outport
  wires:
  In/1 -> Compare To Constant1/1, Compare To Constant2/1, Compare To Constant/1
  Compare To Constant1/1 -> Switch/2
  Compare To Constant/1 -> Switch2/2
  Compare To Constant2/1 -> Switch1/2
  Metall/1 -> Switch1/1
  Schwarz/1 -> Switch/1
  Weiss(Gelb)/1 -> Switch2/1
  Constant/1 -> Switch2/3
  Constant2/1 -> Switch/3
  Constant1/1 -> Switch1/3
  Switch/1 -> MinMax/2
  Switch2/1 -> MinMax/1
  Switch1/1 -> MinMax/3
  MinMax/1 -> Out/1

== system Scenario_13_CoDeSys/Stempelanlage/BT_7_Farbe ==
  In : Inport
  Compare To Constant : simulink/Logic and Bit Operations/Compare To Constant  relop===  const=0  OutDataTypeStr=boolean
  Compare To Constant1 : simulink/Logic and Bit Operations/Compare To Constant  relop===  const=1  OutDataTypeStr=boolean
  Compare To Constant2 : simulink/Logic and Bit Operations/Compare To Constant  relop===  const=2  OutDataTypeStr=boolean
  Constant : Constant  Value=[0 0 0]
  Constant1 : Constant  Value=[0 0 0]
  Constant2 : Constant  Value=[0 0 0]
  Metall : Constant  Value=Bauteil_Farbe_Metall
  MinMax : MinMax  Function=max  Inputs=3
  Schwarz : Constant  Value=Bauteil_Farbe_Schwarz
  Switch : Switch  Threshold=1
  Switch1 : Switch  Threshold=1
  Switch2 : Switch  Threshold=1
  Weiss(Gelb) : Constant  Value=Bauteil_Farbe_Weiss
  Out : Outport
  wires:
  In/1 -> Compare To Constant1/1, Compare To Constant2/1, Compare To Constant/1
  Compare To Constant1/1 -> Switch/2
  Compare To Constant/1 -> Switch2/2
  Compare To Constant2/1 -> Switch1/2
  Metall/1 -> Switch1/1
  Schwarz/1 -> Switch/1
  Weiss(Gelb)/1 -> Switch2/1
  Constant/1 -> Switch2/3
  Constant2/1 -> Switch/3
  Constant1/1 -> Switch1/3
  Switch/1 -> MinMax/2
  Switch2/1 -> MinMax/1
  Switch1/1 -> MinMax/3
  MinMax/1 -> Out/1

== system Scenario_13_CoDeSys/Stempelanlage/BT_8_Farbe ==
  In : Inport
  Compare To Constant : simulink/Logic and Bit Operations/Compare To Constant  relop===  const=0  OutDataTypeStr=boolean
  Compare To Constant1 : simulink/Logic and Bit Operations/Compare To Constant  relop===  const=1  OutDataTypeStr=boolean
  Compare To Constant2 : simulink/Logic and Bit Operations/Compare To Constant  relop===  const=2  OutDataTypeStr=boolean
  Constant : Constant  Value=[0 0 0]
  Constant1 : Constant  Value=[0 0 0]
  Constant2 : Constant  Value=[0 0 0]
  Metall : Constant  Value=Bauteil_Farbe_Metall
  MinMax : MinMax  Function=max  Inputs=3
  Schwarz : Constant  Value=Bauteil_Farbe_Schwarz
  Switch : Switch  Threshold=1
  Switch1 : Switch  Threshold=1
  Switch2 : Switch  Threshold=1
  Weiss(Gelb) : Constant  Value=Bauteil_Farbe_Weiss
  Out : Outport
  wires:
  In/1 -> Compare To Constant1/1, Compare To Constant2/1, Compare To Constant/1
  Compare To Constant1/1 -> Switch/2
  Compare To Constant/1 -> Switch2/2
  Compare To Constant2/1 -> Switch1/2
  Metall/1 -> Switch1/1
  Schwarz/1 -> Switch/1
  Weiss(Gelb)/1 -> Switch2/1
  Constant/1 -> Switch2/3
  Constant2/1 -> Switch/3
  Constant1/1 -> Switch1/3
  Switch/1 -> MinMax/2
  Switch2/1 -> MinMax/1
  Switch1/1 -> MinMax/3
  MinMax/1 -> Out/1

== system Scenario_13_CoDeSys/Stempelanlage/BT_9_Farbe ==
  In : Inport
  Compare To Constant : simulink/Logic and Bit Operations/Compare To Constant  relop===  const=0  OutDataTypeStr=boolean
  Compare To Constant1 : simulink/Logic and Bit Operations/Compare To Constant  relop===  const=1  OutDataTypeStr=boolean
  Compare To Constant2 : simulink/Logic and Bit Operations/Compare To Constant  relop===  const=2  OutDataTypeStr=boolean
  Constant : Constant  Value=[0 0 0]
  Constant1 : Constant  Value=[0 0 0]
  Constant2 : Constant  Value=[0 0 0]
  Metall : Constant  Value=Bauteil_Farbe_Metall
  MinMax : MinMax  Function=max  Inputs=3
  Schwarz : Constant  Value=Bauteil_Farbe_Schwarz
  Switch : Switch  Threshold=1
  Switch1 : Switch  Threshold=1
  Switch2 : Switch  Threshold=1
  Weiss(Gelb) : Constant  Value=Bauteil_Farbe_Weiss
  Out : Outport
  wires:
  In/1 -> Compare To Constant1/1, Compare To Constant2/1, Compare To Constant/1
  Compare To Constant1/1 -> Switch/2
  Compare To Constant/1 -> Switch2/2
  Compare To Constant2/1 -> Switch1/2
  Metall/1 -> Switch1/1
  Schwarz/1 -> Switch/1
  Weiss(Gelb)/1 -> Switch2/1
  Constant/1 -> Switch2/3
  Constant2/1 -> Switch/3
  Constant1/1 -> Switch1/3
  Switch/1 -> MinMax/2
  Switch2/1 -> MinMax/1
  Switch1/1 -> MinMax/3
  MinMax/1 -> Out/1

== system Scenario_13_CoDeSys/Stempelanlage/Band_Lampen_Switch ==
  Lampe_Gruen_In : Inport
  Lampe_Rot_In : Inport  Port=2
  Compare To Constant1 : simulink/Logic and Bit Operations/Compare To Constant  relop===  const=1  OutDataTypeStr=boolean
  Compare To Constant2 : simulink/Logic and Bit Operations/Compare To Constant  relop=>=  const=0.5  OutDataTypeStr=boolean
  Compare To Constant3 : simulink/Logic and Bit Operations/Compare To Constant  relop=<=  const=0.8  OutDataTypeStr=boolean
  Compare To Constant4 : simulink/Logic and Bit Operations/Compare To Constant  relop=<=  const=0.2  OutDataTypeStr=boolean
  Compare To Constant5 : simulink/Logic and Bit Operations/Compare To Constant  relop=>=  const=-0.2  OutDataTypeStr=boolean
  Compare To Constant6 : simulink/Logic and Bit Operations/Compare To Constant  relop=<=  const=5.9  OutDataTypeStr=boolean
  Compare To Constant7 : simulink/Logic and Bit Operations/Compare To Constant  relop=>=  const=3.3  OutDataTypeStr=boolean
  Constant : Constant  Value=[0, 0.8, 0]
  Constant1 : Constant  Value=[0.8, 0.8, 0.8]
  Constant2 : Constant  Value=[1, 0, 0]
  Constant3 : Constant  Value=[0.8, 0.8, 0.8]
  Logical Operator1 : Logic  Inputs=4  AllPortsSameDT=off  OutDataTypeStr=boolean
  Logical Operator2 : Logic  AllPortsSameDT=off  OutDataTypeStr=boolean
  Logical Operator3 : Logic  AllPortsSameDT=off  OutDataTypeStr=boolean
  Logical Operator4 : Logic  AllPortsSameDT=off  OutDataTypeStr=boolean
  Switch : Switch  Threshold=1
  Switch1 : Switch  Threshold=1
  Lampe_Gruen_Out : Outport
  Lampe_Rot_Out : Outport  Port=2
  wires:
  Compare To Constant2/1 -> Logical Operator3/1
  Compare To Constant3/1 -> Logical Operator3/2
  Compare To Constant1/1 -> Logical Operator1/1
  Logical Operator3/1 -> Logical Operator1/2
  Compare To Constant4/1 -> Logical Operator2/1
  Compare To Constant5/1 -> Logical Operator2/2
  Logical Operator2/1 -> Logical Operator1/3
  Compare To Constant6/1 -> Logical Operator4/1
  Compare To Constant7/1 -> Logical Operator4/2
  Logical Operator4/1 -> Logical Operator1/4
  Lampe_Gruen_In/1 -> Switch/2
  Switch/1 -> Lampe_Gruen_Out/1
  Constant/1 -> Switch/1
  Constant1/1 -> Switch/3
  Switch1/1 -> Lampe_Rot_Out/1
  Constant2/1 -> Switch1/1
  Constant3/1 -> Switch1/3
  Lampe_Rot_In/1 -> Switch1/2

== system Scenario_13_CoDeSys/Stempelanlage/Lager_Lampen_Switch ==
  Lampe_Gruen_In : Inport
  Lampe_Rot_In : Inport  Port=2
  Constant : Constant  Value=[0, 0.8, 0]
  Constant1 : Constant  Value=[0.8, 0.8, 0.8]
  Constant2 : Constant  Value=[1, 0, 0]
  Constant3 : Constant  Value=[0.8, 0.8, 0.8]
  Switch : Switch  Threshold=1
  Switch1 : Switch  Threshold=1
  Lampe_Gruen_Out : Outport
  Lampe_Rot_Out : Outport  Port=2
  wires:
  Lampe_Gruen_In/1 -> Switch/2
  Switch/1 -> Lampe_Gruen_Out/1
  Constant/1 -> Switch/1
  Constant1/1 -> Switch/3
  Switch1/1 -> Lampe_Rot_Out/1
  Constant2/1 -> Switch1/1
  Constant3/1 -> Switch1/3
  Lampe_Rot_In/1 -> Switch1/2

== system Scenario_13_CoDeSys/Stempelanlage/Stempel_Lampen_Switch ==
  Lampe_Gruen_In : Inport
  Lampe_Rot_In : Inport  Port=2
  Compare To Constant1 : simulink/Logic and Bit Operations/Compare To Constant  relop===  const=1  OutDataTypeStr=boolean
  Compare To Constant2 : simulink/Logic and Bit Operations/Compare To Constant  relop=>=  const=0.5  OutDataTypeStr=boolean
  Compare To Constant3 : simulink/Logic and Bit Operations/Compare To Constant  relop=<=  const=0.8  OutDataTypeStr=boolean
  Compare To Constant4 : simulink/Logic and Bit Operations/Compare To Constant  relop=<=  const=0.2  OutDataTypeStr=boolean
  Compare To Constant5 : simulink/Logic and Bit Operations/Compare To Constant  relop=>=  const=-0.2  OutDataTypeStr=boolean
  Compare To Constant6 : simulink/Logic and Bit Operations/Compare To Constant  relop=<=  const=5.9  OutDataTypeStr=boolean
  Compare To Constant7 : simulink/Logic and Bit Operations/Compare To Constant  relop=>=  const=3.3  OutDataTypeStr=boolean
  Constant : Constant  Value=[0, 0.8, 0]
  Constant1 : Constant  Value=[0.8, 0.8, 0.8]
  Constant2 : Constant  Value=[1, 0, 0]
  Constant3 : Constant  Value=[0.8, 0.8, 0.8]
  Logical Operator1 : Logic  Inputs=4  AllPortsSameDT=off  OutDataTypeStr=boolean
  Logical Operator2 : Logic  AllPortsSameDT=off  OutDataTypeStr=boolean
  Logical Operator3 : Logic  AllPortsSameDT=off  OutDataTypeStr=boolean
  Logical Operator4 : Logic  AllPortsSameDT=off  OutDataTypeStr=boolean
  Switch : Switch  Threshold=1
  Switch1 : Switch  Threshold=1
  Lampe_Gruen_Out : Outport
  Lampe_Rot_Out : Outport  Port=2
  wires:
  Compare To Constant2/1 -> Logical Operator3/1
  Compare To Constant3/1 -> Logical Operator3/2
  Compare To Constant1/1 -> Logical Operator1/1
  Logical Operator3/1 -> Logical Operator1/2
  Compare To Constant4/1 -> Logical Operator2/1
  Compare To Constant5/1 -> Logical Operator2/2
  Logical Operator2/1 -> Logical Operator1/3
  Compare To Constant6/1 -> Logical Operator4/1
  Compare To Constant7/1 -> Logical Operator4/2
  Logical Operator4/1 -> Logical Operator1/4
  Lampe_Gruen_In/1 -> Switch/2
  Switch/1 -> Lampe_Gruen_Out/1
  Constant/1 -> Switch/1
  Constant1/1 -> Switch/3
  Switch1/1 -> Lampe_Rot_Out/1
  Constant2/1 -> Switch1/1
  Constant3/1 -> Switch1/3
  Lampe_Rot_In/1 -> Switch1/2
